simulink model "Sim_Prob2"  (R2017b)
settings: Solver=FixedStepAuto  StartTime=0.0  StopTime=20.0  FixedStep=0.001  RelTol=1e-3
undefined symbols (not defined in the file or in its folder): K
settings Model: Creator=Daslab  LastModifiedBy=Daslab

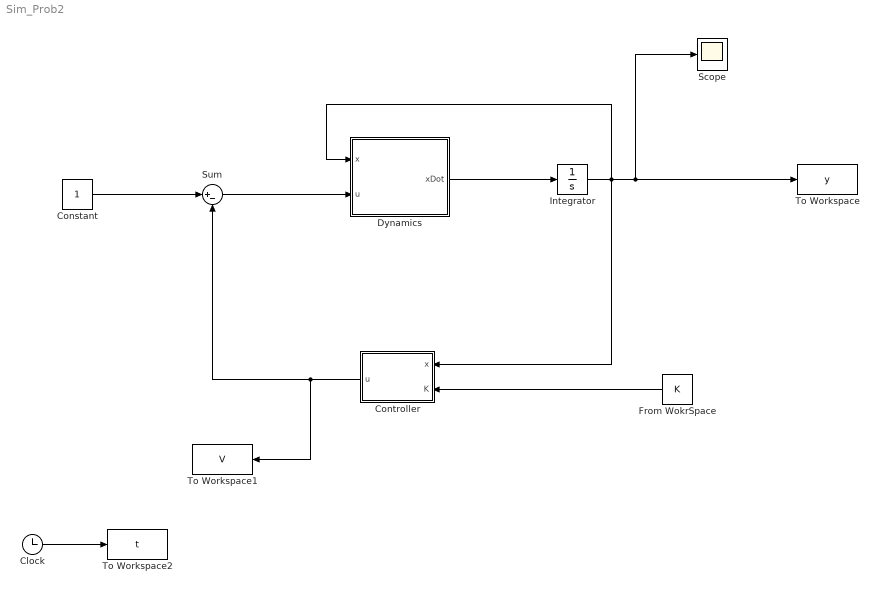
== system Sim_Prob2 ==
  Clock : Clock
  Constant : Constant
  Controller : MATLAB Function  TreatAsAtomicUnit=on
  Dynamics : MATLAB Function  TreatAsAtomicUnit=on
  From WokrSpace : Constant  Value=K
  Integrator : Integrator  InitialCondition=[0;0;0]
  Scope : Scope
  Sum : Sum  Inputs=|+-
  To Workspace : ToWorkspace  VariableName=y  SampleTime=-1
      settings: Save2DSignal=2-D array (concatenate along first dimension)
  To Workspace1 : ToWorkspace  VariableName=V  SampleTime=-1
      settings: Save2DSignal=2-D array (concatenate along first dimension)
  To Workspace2 : ToWorkspace  VariableName=t  SampleTime=-1
      settings: Save2DSignal=2-D array (concatenate along first dimension)
  wires:
  Dynamics/1(xDot) -> Integrator/1
  Integrator/1 -> Controller/1(x), Dynamics/1(x), Scope/1, To Workspace/1
  Controller/1(u) -> To Workspace1/1, Sum/2
  From WokrSpace/1 -> Controller/2(K)
  Constant/1 -> Sum/1
  Sum/1 -> Dynamics/2(u)
  Clock/1 -> To Workspace2/1

== matlab function Sim_Prob2/Controller ==
  data: x input; u output; K input
function u = Controller(x,K)

u = K'*x;

== matlab function Sim_Prob2/Dynamics ==
  data: x input; u input; xDot output
function xDot = Dynamics(x,u)

Lp = -1; % rad/s
Ldela = 30; % s^-2; 
tau = 0.1; % sec 
% 
% Deldela_max = 0.436; % rad 
% Delphi_max = 0.787; % rad 
% delv_max = 10; % volts

A = [Lp 0 Ldela; 
     1  0 0; 
     0  0 -1/tau];

B = [0 0 1/tau]';

xDot = A*x + B*u;
